simulink model "MPC_Omkar_2018"  (R2018b)
settings: Solver=ode45  StartTime=0.0  StopTime=0.05  FixedStep=10e-6  RelTol=1e-3
InitFcn:
  | Ts=100e-6;
libraries: powerlib x14, simulink x2, pePwmGenerator x1, powerlib_meascontrol x1
settings Model: Creator=zero  LastModifiedBy=zero
settings SolverCC: AlgebraicLoopSolver=LineSearch

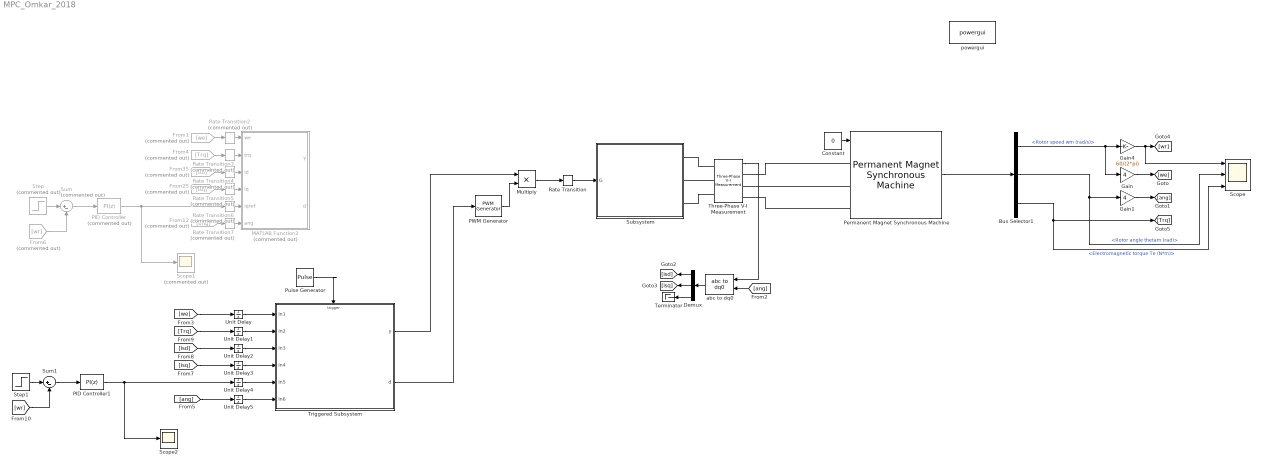
== system MPC_Omkar_2018 ==
  Bus Selector1 : BusSelector  OutputSignals=Rotor speed wm (rad/s),Rotor angle thetam (rad),Electromagnetic torque Te (N*m)
  Constant : Constant  Value=0
  Demux : Demux  Outputs=3
  From1 : From  Commented=on  GotoTag=we
  From12 : From  Commented=on  GotoTag=ang
  From25 : From  Commented=on  GotoTag=isq
  From35 : From  Commented=on  GotoTag=isd
  From4 : From  Commented=on  GotoTag=Trq
  From6 : From  Commented=on  GotoTag=wr
  Gain : Gain  Gain=4  SaturateOnIntegerOverflow=on  OutDataTypeStr=Inherit: Same as input  ParamDataTypeStr=Inherit: Same as input
  Gain1 : Gain  Gain=4  SaturateOnIntegerOverflow=on  OutDataTypeStr=Inherit: Same as input  ParamDataTypeStr=Inherit: Same as input
  Gain4 : Gain  Gain=60/(2*pi)  SaturateOnIntegerOverflow=on  OutDataTypeStr=Inherit: Same as input  ParamDataTypeStr=Inherit: Same as input
  MATLAB Function2 : MATLAB Function  Commented=on  TreatAsAtomicUnit=on
  Multiply : Product
  PID Controller : simulink/Continuous/PID Controller  Commented=on  Controller=PI  Form=Parallel  TimeDomain=Discrete-time  SampleTime=Ts  IntegratorMethod=Forward Euler  FilterMethod=Forward Euler  ControllerParametersSource=internal  P=2  I=0.1  D=5  UseFilter=on  N=100  TunerSelectOption=Transfer Function Based (PID Tuner App)  InitialConditionSource=internal  InitialConditionForIntegrator=0  InitialConditionForFilter=0  DifferentiatorICPrevScaledInput=0  ExternalReset=none  TrackingMode=off  Kt=1  LimitOutput=on  UpperSaturationLimit=3  LowerSaturationLimit=-3  LinearizeAsGain=on  AntiWindupMode=clamping  Kb=1  POutMin=[]  POutMax=[]  IOutMin=[]  IOutMax=[]  DOutMin=[]  DOutMax=[]  NOutMin=[]  NOutMax=[]  SumOutMin=[]  SumOutMax=[]  SaturationOutMin=[]  SaturationOutMax=[]  PParamMin=[]  PParamMax=[]  IParamMin=[]  IParamMax=[]  DParamMin=[]  DParamMax=[]  NParamMin=[]  NParamMax=[]  KbParamMin=[]  KbParamMax=[]  KtParamMin=[]  KtParamMax=[]  KbOutMin=[]  KbOutMax=[]  KtOutMin=[]  KtOutMax=[]  IntegratorOutMin=[]  IntegratorOutMax=[]  FilterOutMin=[]  FilterOutMax=[]  SumI1OutMin=[]  SumI1OutMax=[]  SumI2OutMin=[]  SumI2OutMax=[]  SumI3OutMin=[]  SumI3OutMax=[]  SumI4OutMin=[]  SumI4OutMax=[]  SumDOutMin=[]  SumDOutMax=[]  DifferentiatorOutMin=[]  DifferentiatorOutMax=[]  FilterDiffOutCoefMin=[]  FilterDiffOutCoefMax=[]  ReciprocalOutMin=[]  ReciprocalOutMax=[]  SumDenOutMin=[]  SumDenOutMax=[]  SumNumOutMin=[]  SumNumOutMax=[]  DivideOutMin=[]  DivideOutMax=[]  IntegratorContinuousStateAttributes=''  IntegratorStateMustResolveToSignalObject=off  IntegratorRTWStateStorageClass=Auto  FilterContinuousStateAttributes=''  FilterStateMustResolveToSignalObject=off  FilterRTWStateStorageClass=Auto  ParallelPVariant=InternalParameters  IdealPVariant=Disabled  IVariant=InternalParameters  DVariant=Disabled  IntegratorVariant=Discrete  SatVariant=Enabled  AWVariant=DiscClampingParallel  PCopyVariant=Disabled  TRVariant=Disabled  FdbkBlocksVariant=Forward  IdealPFdbkVariant=Disabled  SatFdbkVariant=Disabled  DerivativeFilterVariant=Disabled  NVariant=Disabled  NCopyVariant=Disabled_SignalSpec  FilterICVariant=Disabled  IntegratorICVariant=InternalICs  ExternalResetVariant=Disabled  TRSumVariant=Passthrough  SumFdbkVariant=Disabled  SumVariant=Sum_PI
  PID Controller1 : simulink/Continuous/PID Controller  Controller=PI  Form=Parallel  TimeDomain=Discrete-time  SampleTime=Ts  IntegratorMethod=Forward Euler  FilterMethod=Forward Euler  ControllerParametersSource=internal  P=0.03  I=0.001  D=5  UseFilter=on  N=100  TunerSelectOption=Transfer Function Based (PID Tuner App)  InitialConditionSource=internal  InitialConditionForIntegrator=0  InitialConditionForFilter=0  DifferentiatorICPrevScaledInput=0  ExternalReset=none  TrackingMode=off  Kt=1  LimitOutput=on  UpperSaturationLimit=3  LowerSaturationLimit=-3  LinearizeAsGain=on  AntiWindupMode=clamping  Kb=1  POutMin=[]  POutMax=[]  IOutMin=[]  IOutMax=[]  DOutMin=[]  DOutMax=[]  NOutMin=[]  NOutMax=[]  SumOutMin=[]  SumOutMax=[]  SaturationOutMin=[]  SaturationOutMax=[]  PParamMin=[]  PParamMax=[]  IParamMin=[]  IParamMax=[]  DParamMin=[]  DParamMax=[]  NParamMin=[]  NParamMax=[]  KbParamMin=[]  KbParamMax=[]  KtParamMin=[]  KtParamMax=[]  KbOutMin=[]  KbOutMax=[]  KtOutMin=[]  KtOutMax=[]  IntegratorOutMin=[]  IntegratorOutMax=[]  FilterOutMin=[]  FilterOutMax=[]  SumI1OutMin=[]  SumI1OutMax=[]  SumI2OutMin=[]  SumI2OutMax=[]  SumI3OutMin=[]  SumI3OutMax=[]  SumI4OutMin=[]  SumI4OutMax=[]  SumDOutMin=[]  SumDOutMax=[]  DifferentiatorOutMin=[]  DifferentiatorOutMax=[]  FilterDiffOutCoefMin=[]  FilterDiffOutCoefMax=[]  ReciprocalOutMin=[]  ReciprocalOutMax=[]  SumDenOutMin=[]  SumDenOutMax=[]  SumNumOutMin=[]  SumNumOutMax=[]  DivideOutMin=[]  DivideOutMax=[]  IntegratorContinuousStateAttributes=''  IntegratorStateMustResolveToSignalObject=off  IntegratorRTWStateStorageClass=Auto  FilterContinuousStateAttributes=''  FilterStateMustResolveToSignalObject=off  FilterRTWStateStorageClass=Auto  ParallelPVariant=InternalParameters  IdealPVariant=Disabled  IVariant=InternalParameters  DVariant=Disabled  IntegratorVariant=Discrete  SatVariant=Enabled  AWVariant=DiscClampingParallel  PCopyVariant=Disabled  TRVariant=Disabled  FdbkBlocksVariant=Forward  IdealPFdbkVariant=Disabled  SatFdbkVariant=Disabled  DerivativeFilterVariant=Disabled  NVariant=Disabled  NCopyVariant=Disabled_SignalSpec  FilterICVariant=Disabled  IntegratorICVariant=InternalICs  ExternalResetVariant=Disabled  TRSumVariant=Passthrough  SumFdbkVariant=Disabled  SumVariant=Sum_PI
  PWM Generator : pePwmGenerator/PWM Generator  CarrCount=Up  Tper=0.001  Ts=5e-5
  Permanent Magnet Synchronous Machine : powerlib/Machines/Permanent Magnet Synchronous Machine  NbPhases=3  FluxDistribution=Sinusoidal  RotorType=Round  MechanicalLoad=Torque Tm  PresetModel=No  ShowDetailedParameters=on  MeasurementBus=off  Resistance=0.375  Inductance=8.5e-3  dqInductances=[8.5e-3,8.5e-3]  La=0.0002  MachineConstant=Flux linkage established by magnets (V.s)  Flux=0.0068916  VoltageCst=5  TorqueCst=0.04135  Flat=120  Mechanical=[2.66e-6 1.3e-6 4 0]  PolePairs=4  InitialConditions=[0,0, 0,0]  InitialConditions5ph=[0 0 0 0 0 0]  TsPowergui=0  TsBlock=-1  RefAngle=90 degrees behind phase A axis (modified Park)
      settings: SourceProductName=Simscape Power Systems
  Pulse Generator : DiscretePulseGenerator  PulseType=Time based  Period=0.00005  PulseWidth=5
  Rate Transition : RateTransition
  Rate Transition{2..7} (6 alike) : RateTransition  Commented=on
  Scope : Scope  NumInputPorts=3
  Scope1 : Scope  Commented=on
  Scope2 : Scope
  Step : Step  Commented=on  Time=0  After=1000  SampleTime=0
  Step1 : Step  Time=0  After=1000  SampleTime=0
  Subsystem : Subsystem
  Sum : Sum  Commented=on  Inputs=|+-
  Sum1 : Sum  Inputs=|+-
  Terminator : Terminator
  Three-Phase V-I Measurement : powerlib/Measurements/Three-Phase V-I Measurement  VoltageMeasurement=no  SetLabelV=off  LabelV=Vabc  Vpu=off  VpuLL=off  CurrentMeasurement=yes  SetLabelI=off  LabelI=Iabc  Ipu=off  Pbase=100e6  Vbase=500e3  OutputType=Complex  PhasorSimulation=off  PSBequivalent=0
  Triggered Subsystem : Subsystem  TreatAsAtomicUnit=on
  Unit Delay{,1..5} (6 alike) : UnitDelay  SampleTime=-1
  abc to dq0 : powerlib_meascontrol/Transformations/abc to dq0  Alignment=90 degrees behind phase A axis
  powergui : powerlib/powergui  Priority=1  SimulationMode=Discrete  SampleTime=1e-7  frequency=60  Iterations=50  frequencyindice=0  Pbase=100e6  ErrMax=1e-4  UnitsV=kV  UnitsW=MW  buscounter=0  FunctionMessages=off  echomessages=off  EnableUseOfTLC=off  CurrentSourceSwitches=off  DisableSnubberDevices=off  DisableRonSwitches=off  DisableVfSwitches=off  DisplayEquations=off  SolverType=Tustin/Backward Euler (TBE)  Interpol=off  ExternalGateDelay=off  methode=off  Ts=100  x0status=blocks  SPID=on  SwTol=0  HookPort=off  RestoreLinks=warning  ResistiveCurrentMeasurement=off  Frange=[0:2:500]  Ylog=off  Xlog=on  ShowGrid=off  save=off  variable=ZData  structure=0  ZoomFFT=off  StartTime=0.0  cycles=1  DisplayStyle=1  fundamental=60  FreqAxis=off  MaxFrequency=1000  frequencyindicesteady=1  RmsSteady=1  display=off
  wires:
  Step/1 -> Sum/1
  From6/1 -> Sum/2
  Permanent Magnet Synchronous Machine/1 -> Bus Selector1/1
  Gain4/1 -> Scope/1, [wr]
  Gain/1 -> [we]
  Gain1/1 -> [ang]
  Bus Selector1/1 -> Gain/1, Gain4/1  "<Rotor speed wm (rad/s)>"
  Bus Selector1/3 -> [Trq], Scope/3  "<Electromagnetic torque Te (N*m)>"
  Bus Selector1/2 -> Scope/2, Gain1/1  "<Rotor angle thetam (rad)>"
  Three-Phase V-I Measurement/1 -> abc to dq0/1
  [ang] -> abc to dq0/2
  abc to dq0/1 -> Demux/1
  Demux/1 -> [isd]
  Demux/2 -> [isq]
  Demux/3 -> Terminator/1
  PWM Generator/1 -> Multiply/2
  Multiply/1 -> Rate Transition/1
  Rate Transition/1 -> Subsystem/1(G)
  Sum/1 -> PID Controller/1
  From1/1 -> Rate Transition2/1
  Rate Transition2/1 -> MATLAB Function2/1(we)
  From4/1 -> Rate Transition3/1
  Rate Transition3/1 -> MATLAB Function2/2(trq)
  From35/1 -> Rate Transition4/1
  Rate Transition4/1 -> MATLAB Function2/3(id)
  From25/1 -> Rate Transition5/1
  Rate Transition5/1 -> MATLAB Function2/4(iq)
  PID Controller/1 -> Scope1/1, Rate Transition6/1
  Rate Transition6/1 -> MATLAB Function2/5(iqref)
  From12/1 -> Rate Transition7/1
  Rate Transition7/1 -> MATLAB Function2/6(ang)
  Constant/1 -> Permanent Magnet Synchronous Machine/1
  [ang] -> Unit Delay5/1
  PID Controller1/1 -> Unit Delay4/1, Scope2/1
  [isq] -> Unit Delay3/1
  [isd] -> Unit Delay2/1
  [Trq] -> Unit Delay1/1
  [we] -> Unit Delay/1
  Sum1/1 -> PID Controller1/1
  [wr] -> Sum1/2
  Step1/1 -> Sum1/1
  Triggered Subsystem/1(y) -> Multiply/1
  Triggered Subsystem/2(d) -> PWM Generator/1
  Pulse Generator/1 -> Triggered Subsystem/Trigger
  Unit Delay/1 -> Triggered Subsystem/1(In1)
  Unit Delay1/1 -> Triggered Subsystem/2(In2)
  Unit Delay2/1 -> Triggered Subsystem/3(In3)
  Unit Delay3/1 -> Triggered Subsystem/4(In4)
  Unit Delay4/1 -> Triggered Subsystem/5(In5)
  Unit Delay5/1 -> Triggered Subsystem/6(In6)
  connections:
  Three-Phase V-I Measurement/LConn2 -- Subsystem/RConn2
  Three-Phase V-I Measurement/LConn1 -- Subsystem/RConn1
  Three-Phase V-I Measurement/LConn3 -- Subsystem/RConn3
  Permanent Magnet Synchronous Machine/LConn3 -- Three-Phase V-I Measurement/RConn3
  Permanent Magnet Synchronous Machine/LConn2 -- Three-Phase V-I Measurement/RConn2
  Permanent Magnet Synchronous Machine/LConn1 -- Three-Phase V-I Measurement/RConn1

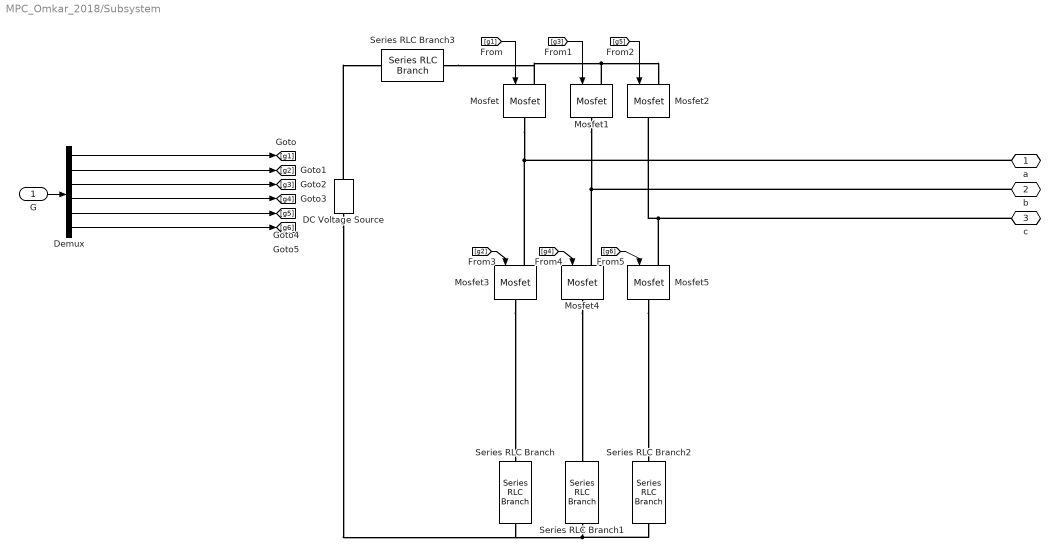
== system MPC_Omkar_2018/Subsystem ==
  G : Inport
  DC Voltage Source : powerlib/Electrical Sources/DC Voltage Source  Amplitude=12  Measurements=None
  Demux : Demux  Outputs=6
  Mosfet{,1..5} (6 alike) : powerlib/Power Electronics/Mosfet  Ron=0.001  Lon=0  Rd=0.0001  Vfd=0  IC=0  Rs=1e5  Cs=inf  Measurements=off
  Series RLC Branch : powerlib/Elements/Series RLC Branch  LConnTagsString=__new0  RConnTagsString=__new0  BranchType=R  Resistance=0.33  Inductance=1e-3  SetiL0=off  InitialCurrent=0  Capacitance=1e-6  Setx0=off  InitialVoltage=0  Measurements=None
  Series RLC Branch1 : powerlib/Elements/Series RLC Branch  LConnTagsString=__new0  RConnTagsString=__new0  BranchType=R  Resistance=0.33  Inductance=1e-3  SetiL0=off  InitialCurrent=0  Capacitance=1e-6  Setx0=off  InitialVoltage=0  Measurements=None
  Series RLC Branch2 : powerlib/Elements/Series RLC Branch  LConnTagsString=__new0  RConnTagsString=__new0  BranchType=R  Resistance=0.33  Inductance=1e-3  SetiL0=off  InitialCurrent=0  Capacitance=1e-6  Setx0=off  InitialVoltage=0  Measurements=None
  Series RLC Branch3 : powerlib/Elements/Series RLC Branch  LConnTagsString=__new0  RConnTagsString=__new0  BranchType=R  Resistance=5  Inductance=1e-3  SetiL0=off  InitialCurrent=0  Capacitance=1e-6  Setx0=off  InitialVoltage=0  Measurements=None
  a : PMIOPort  Side=Right
  b : PMIOPort  Port=2  Side=Right
  c : PMIOPort  Port=3  Side=Right
  wires:
  [g3] -> Mosfet1/1
  [g4] -> Mosfet4/1
  [g2] -> Mosfet3/1
  [g6] -> Mosfet5/1
  [g5] -> Mosfet2/1
  [g1] -> Mosfet/1
  Demux/5 -> [g5]
  G/1 -> Demux/1
  Demux/3 -> [g3]
  Demux/1 -> [g1]
  Demux/2 -> [g2]
  Demux/4 -> [g4]
  Demux/6 -> [g6]
  connections:
  a/RConn1 -- Mosfet3/LConn1 -- Mosfet/RConn1
  b/RConn1 -- Mosfet4/LConn1 -- Mosfet1/RConn1
  c/RConn1 -- Mosfet5/LConn1 -- Mosfet2/RConn1
  Mosfet/LConn1 -- Series RLC Branch3/LConn1 -- Mosfet2/LConn1 -- Mosfet1/LConn1
  Mosfet4/RConn1 -- Series RLC Branch1/LConn1
  Mosfet5/RConn1 -- Series RLC Branch2/LConn1
  DC Voltage Source/LConn1 -- Series RLC Branch/RConn1 -- Series RLC Branch2/RConn1 -- Series RLC Branch1/RConn1
  Mosfet3/RConn1 -- Series RLC Branch/LConn1
  DC Voltage Source/RConn1 -- Series RLC Branch3/RConn1

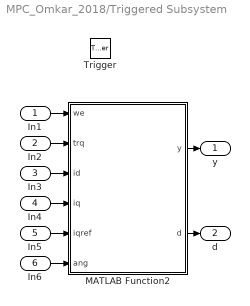
== system MPC_Omkar_2018/Triggered Subsystem ==
  In1 : Inport
  In2 : Inport  Port=2
  In3 : Inport  Port=3
  In4 : Inport  Port=4
  In5 : Inport  Port=5
  In6 : Inport  Port=6
  Trigger : TriggerPort  VariantControl=Variant
  MATLAB Function2 : MATLAB Function  TreatAsAtomicUnit=on
  y : Outport
  d : Outport  Port=2
  wires:
  MATLAB Function2/1(y) -> y/1
  MATLAB Function2/2(d) -> d/1
  In1/1 -> MATLAB Function2/1(we)
  In2/1 -> MATLAB Function2/2(trq)
  In3/1 -> MATLAB Function2/3(id)
  In4/1 -> MATLAB Function2/4(iq)
  In5/1 -> MATLAB Function2/5(iqref)
  In6/1 -> MATLAB Function2/6(ang)

== matlab function MPC_Omkar_2018/Triggered Subsystem/MATLAB Function2 ==
  data: y output; we input; trq input; id input; iq input; iqref input; ang input; d output
function [y,d]  = MPC(we,trq, id,iq,iqref,ang)

persistent oldState;

if isempty(oldState)
    oldState = 1;
end

Ts = 50e-6;
Vdc = 12;
L = 0.0002;
R = 0.375;
psiPM = 0.0068916;

c = 0.2;
p = 0.4;
k = 0.6;
g = 0.8;

states =[0.9 0     0 0.9     0 0.9;
         0.9 0     0.9 0     0 0.9;
         0 0.9     0.9 0     0 0.9;
         0 0.9     0.9 0     0.9 0;
         0 0.9     0 0.9     0.9 0;
         0.9 0     0 0.9     0.9 0;
         0.5 0     0 0.5     0 0.5;
        0.5 0     0.5 0     0 0.5;
        0 0.5     0.5 0     0 0.5;
        0 0.5     0.5 0     0.5 0;
        0 0.5     0 0.5     0.5 0;
        0.5 0     0 0.5     0.5 0;];

y = states(1,:)';
cost = [];

for i=1:length(states)
    vsd = (2*Vdc/3)*[sin(ang) sin(ang - (2*pi/3)) sin(ang + (2*pi/3))]*states(i,[1,3,5])';
    vsq = (2*Vdc/3)*[cos(ang) cos(ang - (2*pi/3)) cos(ang + (2*pi/3))]*states(i,[1,3,5])';
    
    id_p = id;
    iq_p = iq;
    
    for x = 1:4
        id_p = ((1-(R*Ts/L))*id_p)+(Ts*we*iq_p)+(vsd*Ts/L);
        iq_p = ((1-(R*Ts/L))*iq_p)-(Ts*we*id_p)-(psiPM*we*Ts)+(vsq*Ts/L);
    end
    
    cost = [cost (id_p)^2 + (iqref - iq_p)^2];
end

a = find(cost == min(cost));
a = a(1);

d = max(states(a,:));

oldState = a;
y = [states(a,:)>0]'*1;

== matlab function MPC_Omkar_2018/MATLAB Function2 ==
  data: y output; we input; trq input; id input; iq input; iqref input; ang input; d output
function [y,d]  = MPC(we,trq, id,iq,iqref,ang)

persistent oldState;

if isempty(oldState)
    oldState = 1;
end

Ts = 100e-6;
Vdc = 12;
L = 0.0002;
R = 0.375;
psiPM = 0.0133;

c = 0.2;
p = 0.4;
k = 0.6;
g = 0.8;

states =[0.9 0     0 0.9     0 0.9;
         0.9 0     0.9 0     0 0.9;
         0 0.9     0.9 0     0 0.9;
         0 0.9     0.9 0     0.9 0;
         0 0.9     0 0.9     0.9 0;
         0.9 0     0 0.9     0.9 0;
         0.5 0     0 0.5     0 0.5;
        0.5 0     0.5 0     0 0.5;
        0 0.5     0.5 0     0 0.5;
        0 0.5     0.5 0     0.5 0;
        0 0.5     0 0.5     0.5 0;
        0.5 0     0 0.5     0.5 0;
        0.25 0     0 0.25     0 0.25;
        0.25 0     0.25 0     0 0.25;
        0 0.25     0.25 0     0 0.25;
        0 0.25     0.25 0     0.25 0;
        0 0.25     0 0.25     0.25 0;
        0.25 0     0 0.25     0.25 0;];

y = states(1,:)';
cost = [];

for i=1:length(states)
    vsd = (2*Vdc/3)*[sin(ang) sin(ang - (2*pi/3)) sin(ang + (2*pi/3))]*states(i,[1,3,5])';
    vsq = (2*Vdc/3)*[cos(ang) cos(ang - (2*pi/3)) cos(ang + (2*pi/3))]*states(i,[1,3,5])';
    
    id_p = id;
    iq_p = iq;
    
    for x = 1:4
        id_p = ((1-(R*Ts/L))*id_p)+(Ts*we*iq_p)+(vsd*Ts/L);
        iq_p = ((1-(R*Ts/L))*iq_p)-(Ts*we*id_p)-(psiPM*we*Ts)+(vsq*Ts/L);
    end
    
    cost = [cost (id_p)^2 + (iqref - iq_p)^2];
end

a = find(cost == min(cost));
a = a(1);

d = max(states(a,:));

oldState = a;
y = [states(a,:)>0]'*1;
